simulink model "FieldControl_PID"  (R2021a)
settings: Solver=ode45  StartTime=0.0  StopTime=3  FixedStep=1e-5  MaxStep=1e-6  RelTol=1e-3
model workspace (MAT data in the model file):
  KI_s = 1
  KP_s = 1
undefined symbols (not defined in the file): DiscIntNeverNeededParam, Fsw, sigbuilder_block
libraries: simulink x2, spspowerguiLib x2
(part 2 of 2)

== system FieldControl_PID/Field_control_PID/Current_control/PMSM/Clark_Transformation ==
  Va : Inport
  Vb : Inport  Port=2
  Vc : Inport  Port=3
  Add : Sum  Inputs=+++
  Add1 : Sum
  Gain : Gain  Gain=-0.5
  Gain1 : Gain  Gain=-0.5
  Gain2 : Gain  Gain=2/3
  Gain3 : Gain  Gain=sqrt(3)/2
  Gain4 : Gain  Gain=-sqrt(3)/2
  Gain5 : Gain  Gain=2/3
  V_alpha : Outport
  V_beta : Outport  Port=2
  wires:
  Gain5/1 -> V_beta/1
  Add1/1 -> Gain5/1
  Gain3/1 -> Add1/1
  Gain4/1 -> Add1/2
  Gain2/1 -> V_alpha/1
  Add/1 -> Gain2/1
  Va/1 -> Add/1
  Gain1/1 -> Add/3
  Gain/1 -> Add/2
  Vc/1 -> Gain1/1, Gain4/1
  Vb/1 -> Gain/1, Gain3/1

== system FieldControl_PID/Field_control_PID/Current_control/PMSM/Electrical_system1 ==
  V_d : Inport
  V_q : Inport  Port=2
  W_e : Inport  Port=3
  Add : Sum  Inputs=-++
  Add1 : Sum  Inputs=+---
  Gain : Gain  Gain=1/Ld
  Gain1 : Gain  Gain=R/Ld
  Gain2 : Gain  Gain=Lq/Ld
  Gain3 : Gain  Gain=1/Lq
  Gain4 : Gain  Gain=R/Lq
  Gain5 : Gain  Gain=Ld/Lq
  Gain6 : Gain  Gain=lamda_pm/Lq
  Integrator : Integrator
  Integrator1 : Integrator
  Product : Product
  Product1 : Product
  I_d : Outport
  I_q : Outport  Port=2
  wires:
  Integrator/1 -> Gain5/1, Gain1/1, I_d/1
  Integrator1/1 -> Gain4/1, Gain2/1, I_q/1
  V_d/1 -> Gain/1
  Gain/1 -> Add/2
  Gain1/1 -> Add/1
  Add/1 -> Integrator/1
  Gain2/1 -> Product/2
  W_e/1 -> Product1/2, Gain6/1, Product/1
  Product/1 -> Add/3
  V_q/1 -> Gain3/1
  Gain3/1 -> Add1/1
  Gain4/1 -> Add1/4
  Gain5/1 -> Product1/1
  Product1/1 -> Add1/2
  Gain6/1 -> Add1/3
  Add1/1 -> Integrator1/1

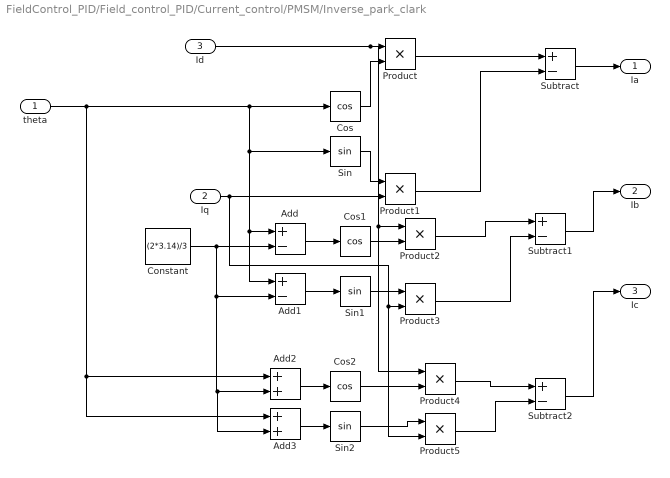
== system FieldControl_PID/Field_control_PID/Current_control/PMSM/Inverse_park_clark ==
  theta : Inport
  Iq : Inport  Port=2
  Id : Inport  Port=3
  Add : Sum  Inputs=+-
  Add1 : Sum  Inputs=+-
  Add2 : Sum
  Add3 : Sum
  Constant : Constant  Value=(2*3.14)/3
  Cos : Trigonometry  Operator=cos
  Cos1 : Trigonometry  Operator=cos
  Cos2 : Trigonometry  Operator=cos
  Product{,1..5} (6 alike) : Product
  Sin : Trigonometry
  Sin1 : Trigonometry
  Sin2 : Trigonometry
  Subtract : Sum  Inputs=+-
  Subtract1 : Sum  Inputs=+-
  Subtract2 : Sum  Inputs=+-
  Ia : Outport
  Ib : Outport  Port=2
  Ic : Outport  Port=3
  wires:
  Add3/1 -> Sin2/1
  Add2/1 -> Cos2/1
  Sin2/1 -> Product5/1
  Cos2/1 -> Product4/2
  Product5/1 -> Subtract2/2
  Product4/1 -> Subtract2/1
  Subtract2/1 -> Ic/1
  Constant/1 -> Add/2, Add1/2, Add2/2, Add3/2
  Subtract1/1 -> Ib/1
  Product3/1 -> Subtract1/2
  Product2/1 -> Subtract1/1
  Sin1/1 -> Product3/1
  Cos1/1 -> Product2/2
  Add1/1 -> Sin1/1
  Add/1 -> Cos1/1
  Product1/1 -> Subtract/2
  Sin/1 -> Product1/1
  Iq/1 -> Product1/2, Product3/2, Product5/2
  Product/1 -> Subtract/1
  Cos/1 -> Product/2
  Id/1 -> Product/1, Product2/1, Product4/1
  theta/1 -> Sin/1, Add/1, Add1/1, Cos/1, Add2/1, Add3/1
  Subtract/1 -> Ia/1

== system FieldControl_PID/Field_control_PID/Current_control/PMSM/Park_Transformation ==
  V_alpha : Inport
  V_beta : Inport  Port=2
  theta : Inport  Port=3
  Add : Sum
  Add1 : Sum
  Cos : Trigonometry  Operator=cos
  Cos1 : Trigonometry
  Gain : Gain  Gain=-1
  Product{,1..3} (4 alike) : Product
  V_d : Outport
  V_q : Outport  Port=2
  wires:
  Add1/1 -> V_q/1
  Product3/1 -> Add1/2
  Gain/1 -> Add1/1
  Product2/1 -> Gain/1
  Add/1 -> V_d/1
  Product1/1 -> Add/2
  Product/1 -> Add/1
  V_beta/1 -> Product1/2, Product3/1
  Cos1/1 -> Product1/1, Product2/2
  Cos/1 -> Product/2, Product3/2
  V_alpha/1 -> Product/1, Product2/1
  theta/1 -> Cos/1, Cos1/1

== system FieldControl_PID/Field_control_PID/Current_control/PMSM/Torque_system ==
  I_d : Inport
  I_q : Inport  Port=2
  Add : Sum  Inputs=+-
  Add1 : Sum
  Constant : Constant  Value=lamda_pm
  Gain : Gain  Gain=(3*P)/4
  Gain1 : Gain  Gain=Ld
  Gain2 : Gain  Gain=Lq
  Product : Product
  Product1 : Product
  Te : Outport
  wires:
  Product1/1 -> Add/2
  Gain2/1 -> Product1/2
  Product/1 -> Add/1
  I_q/1 -> Product/1, Gain2/1
  Add1/1 -> Product/2
  Gain1/1 -> Add1/1
  Constant/1 -> Add1/2
  I_d/1 -> Gain1/1, Product1/1
  Gain/1 -> Te/1
  Add/1 -> Gain/1

== system FieldControl_PID/Field_control_PID/Current_control/SVM-DPWM/Square_signal_generator ==
  Mode : Inport
  F : Inport  Port=2
  If : If  IfExpression=u1 == 1  ElseIfExpressions=u1==2  ShowElse=off
  If Action Subsystem : Subsystem  TreatAsAtomicUnit=on
  If Action Subsystem1 : Subsystem  TreatAsAtomicUnit=on
  Merge : Merge
  Output : Outport
  wires:
  Mode/1 -> If/1
  If/1 -> If Action Subsystem/Action
  F/1 -> If Action Subsystem1/1(F), If Action Subsystem/1(F)
  If/2 -> If Action Subsystem1/Action
  If Action Subsystem/1(out) -> Merge/1
  If Action Subsystem1/1(out) -> Merge/2
  Merge/1 -> Output/1

== system FieldControl_PID/Field_control_PID/Current_control/SVM-DPWM/Variant Subsystem ==
  note: 1) Add Subsystem or Model blocks as valid variant choices.
      | 2) You cannot connect blocks at this level. At simulation, connectivity is automatically
      | determined, based on the active variant and port name matching.
  Va : Inport
  Vb : Inport  Port=2
  Vc : Inport  Port=3
  Iabc : Inport  Port=4
  mag : Inport  Port=5
  Auto : Subsystem  VariantControl=PWM_Mode==3
  DPWM : Subsystem  VariantControl=PWM_Mode==2
  SVM : Subsystem  VariantControl=PWM_Mode==1
  V0 : Outport
  Va* : Outport  Port=2
  Vb* : Outport  Port=3
  Vc* : Outport  Port=4
  PWM_Gen_Mode : Outport  Port=5

== system FieldControl_PID/Field_control_PID/Current_control/Triggered Current Control/FFW ==
  Iq : Inport
  We : Inport  Port=2
  Id : Inport  Port=3
  Add : Sum
  Ld : Gain  Gain=0.0057
  Lq : Gain  Gain=0.0125
  Product : Product
  Product1 : Product
  "delta_pm " : Constant  Value=0.123
  Vq_FFW : Outport
  Vd_FFW : Outport  Port=2
  wires:
  "delta_pm "/1 -> Add/2
  Add/1 -> Product1/1
  Ld/1 -> Add/1
  Id/1 -> Ld/1
  Product1/1 -> Vq_FFW/1
  Product/1 -> Vd_FFW/1
  Lq/1 -> Product/2  "We*Lq"
  We/1 -> Lq/1, Product1/2
  Iq/1 -> Product/1  "Iq"

== system FieldControl_PID/Field_control_PID/Current_control/Triggered Current Control/PID_2 ==
  e : Inport
  Fsw_out : Inport  Port=2
  Discrete-Time Integrator : DiscreteIntegrator  SampleTime=-1  ICPrevOutput=DiscIntNeverNeededParam  ICPrevScaledInput=DiscIntNeverNeededParam
  Gain : Gain
  KI : Gain  Gain=1.2
  Kp : Gain  Gain=0.0125
  Product : Product
  Product1 : Product
  Scope : Scope
  Sum : Sum  Inputs=|++
  v : Outport
  wires:
  e/1 -> KI/1, Kp/1
  Discrete-Time Integrator/1 -> Scope/1, Sum/1
  Sum/1 -> v/1
  KI/1 -> Product/2
  Product/1 -> Discrete-Time Integrator/1
  Fsw_out/1 -> Gain/1
  Kp/1 -> Product1/2
  Product1/1 -> Sum/2
  Gain/1 -> Product1/1, Product/1

== system FieldControl_PID/Field_control_PID/Current_control/Triggered Current Control/PID_3 ==
  Fsw_out : Inport
  e : Inport  Port=2
  Discrete-Time Integrator : DiscreteIntegrator  SampleTime=-1  ICPrevOutput=DiscIntNeverNeededParam  ICPrevScaledInput=DiscIntNeverNeededParam
  Gain : Gain
  KI : Gain  Gain=1.2
  Kp : Gain  Gain=0.0057
  Product : Product
  Product1 : Product
  Sum : Sum  Inputs=|++
  v : Outport
  wires:
  Kp/1 -> Product1/2
  Product1/1 -> Sum/2
  KI/1 -> Product/2
  Product/1 -> Discrete-Time Integrator/1
  e/1 -> KI/1, Kp/1
  Sum/1 -> v/1
  Fsw_out/1 -> Gain/1
  Discrete-Time Integrator/1 -> Sum/1
  Gain/1 -> Product1/1, Product/1

== system FieldControl_PID/Field_control_PID/Current_control/Triggered Current Control/Signal Builder1 ==
  Demux : Demux  Tag=STV Demux  Outputs=1
      settings: DisplayOption=none
  FromWs : FromWorkspace  Tag=STV FromWs  VariableName=tuvar  SampleTime=-1
      SigBuilderData=|
      | common.afterFinalStr = 'Extrapolate'
      | common.sampleTime = '-1'
      | dataSet.timeRange = [0 3]
      | dataSet.name = 'Group 1'
      | sbobj.Groups.Name = 'Group 1'
      | sbobj.Groups.Signals.Name = 'Signal 1'
      | sbobj.Groups.Signals.XData = [0 1 1.5 2 2.5 3]
      | sbobj.Groups.Signals.YData = [2.5 2.5 3.5 3.5 5 5]
      | sbobj.Groups.TimeRange = [0 3]
  Signal 1 : Outport  Tag=STV Outport
  wires:
  Demux/1 -> Signal 1/1
  FromWs/1 -> Demux/1

== system FieldControl_PID/Field_control_PID/Speed_control/Inverse_park_clark/Subsystem ==
  Vd : Inport
  Vq : Inport  Port=2
  Add : Sum
  Square : Math  Operator=square  SaturateOnIntegerOverflow=on
  Square Root : Sqrt  SaturateOnIntegerOverflow=on
  Square1 : Math  Operator=square  SaturateOnIntegerOverflow=on
  Out1 : Outport
  wires:
  Square1/1 -> Add/1
  Add/1 -> Square Root/1
  Vd/1 -> Square1/1
  Square/1 -> Add/2
  Square Root/1 -> Out1/1
  Vq/1 -> Square/1

== system FieldControl_PID/Field_control_PID/Speed_control/PMSM/Clark_Transformation ==
  Va : Inport
  Vb : Inport  Port=2
  Vc : Inport  Port=3
  Add : Sum  Inputs=+++
  Add1 : Sum
  Gain : Gain  Gain=-0.5
  Gain1 : Gain  Gain=-0.5
  Gain2 : Gain  Gain=2/3
  Gain3 : Gain  Gain=sqrt(3)/2
  Gain4 : Gain  Gain=-sqrt(3)/2
  Gain5 : Gain  Gain=2/3
  V_alpha : Outport
  V_beta : Outport  Port=2
  wires:
  Gain5/1 -> V_beta/1
  Add1/1 -> Gain5/1
  Gain3/1 -> Add1/1
  Gain4/1 -> Add1/2
  Gain2/1 -> V_alpha/1
  Add/1 -> Gain2/1
  Va/1 -> Add/1
  Gain1/1 -> Add/3
  Gain/1 -> Add/2
  Vc/1 -> Gain1/1, Gain4/1
  Vb/1 -> Gain/1, Gain3/1

== system FieldControl_PID/Field_control_PID/Speed_control/PMSM/Electrical_system2 ==
  V_d : Inport
  V_q : Inport  Port=2
  W_e : Inport  Port=3
  Add : Sum  Inputs=-++
  Add1 : Sum  Inputs=+---
  Gain : Gain  Gain=1/Ld
  Gain1 : Gain  Gain=R/Ld
  Gain2 : Gain  Gain=Lq/Ld
  Gain3 : Gain  Gain=1/Lq
  Gain4 : Gain  Gain=R/Lq
  Gain5 : Gain  Gain=Ld/Lq
  Gain6 : Gain  Gain=lamda_pm/Lq
  Integrator : Integrator
  Integrator1 : Integrator
  Product : Product
  Product1 : Product
  I_d : Outport
  I_q : Outport  Port=2
  wires:
  Integrator/1 -> Gain5/1, Gain1/1, I_d/1
  Integrator1/1 -> Gain4/1, Gain2/1, I_q/1
  V_d/1 -> Gain/1
  Gain/1 -> Add/2
  Gain1/1 -> Add/1
  Add/1 -> Integrator/1
  Gain2/1 -> Product/2
  W_e/1 -> Gain6/1, Product1/2, Product/1
  Product/1 -> Add/3
  V_q/1 -> Gain3/1
  Gain3/1 -> Add1/1
  Gain4/1 -> Add1/4
  Gain5/1 -> Product1/1
  Product1/1 -> Add1/2
  Gain6/1 -> Add1/3
  Add1/1 -> Integrator1/1

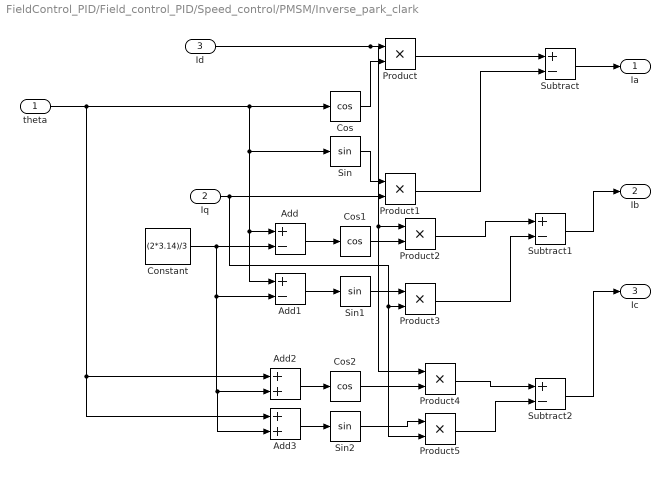
== system FieldControl_PID/Field_control_PID/Speed_control/PMSM/Inverse_park_clark ==
  theta : Inport
  Iq : Inport  Port=2
  Id : Inport  Port=3
  Add : Sum  Inputs=+-
  Add1 : Sum  Inputs=+-
  Add2 : Sum
  Add3 : Sum
  Constant : Constant  Value=(2*3.14)/3
  Cos : Trigonometry  Operator=cos
  Cos1 : Trigonometry  Operator=cos
  Cos2 : Trigonometry  Operator=cos
  Product{,1..5} (6 alike) : Product
  Sin : Trigonometry
  Sin1 : Trigonometry
  Sin2 : Trigonometry
  Subtract : Sum  Inputs=+-
  Subtract1 : Sum  Inputs=+-
  Subtract2 : Sum  Inputs=+-
  Ia : Outport
  Ib : Outport  Port=2
  Ic : Outport  Port=3
  wires:
  Add3/1 -> Sin2/1
  Add2/1 -> Cos2/1
  Sin2/1 -> Product5/1
  Cos2/1 -> Product4/2
  Product5/1 -> Subtract2/2
  Product4/1 -> Subtract2/1
  Subtract2/1 -> Ic/1
  Constant/1 -> Add/2, Add1/2, Add2/2, Add3/2
  Subtract1/1 -> Ib/1
  Product3/1 -> Subtract1/2
  Product2/1 -> Subtract1/1
  Sin1/1 -> Product3/1
  Cos1/1 -> Product2/2
  Add1/1 -> Sin1/1
  Add/1 -> Cos1/1
  Product1/1 -> Subtract/2
  Sin/1 -> Product1/1
  Iq/1 -> Product1/2, Product3/2, Product5/2
  Product/1 -> Subtract/1
  Cos/1 -> Product/2
  Id/1 -> Product/1, Product2/1, Product4/1
  theta/1 -> Sin/1, Add/1, Add1/1, Cos/1, Add2/1, Add3/1
  Subtract/1 -> Ia/1

== system FieldControl_PID/Field_control_PID/Speed_control/PMSM/Mechanical_system ==
  Te : Inport
  Add : Sum  Inputs=+--
  Add1 : Sum
  Gain : Gain  Gain=1/J
  Gain1 : Gain  Gain=1/J
  Gain2 : Gain  Gain=b/J
  Integrator : Integrator
  Step : Step  Time=1.2  Before=0.75  After=0.75  SampleTime=0
  Step1 : Step  Time=1.2  After=0.5  SampleTime=0
  TL : Constant  Value=TL
  Wm : Outport
  wires:
  Gain2/1 -> Add/3
  Gain/1 -> Add/1
  Add/1 -> Integrator/1
  Te/1 -> Gain/1
  Gain1/1 -> Add/2
  Integrator/1 -> Gain2/1, Wm/1
  Add1/1 -> Gain1/1
  Step/1 -> Add1/1
  Step1/1 -> Add1/2

== system FieldControl_PID/Field_control_PID/Speed_control/PMSM/Park_Transformation ==
  V_alpha : Inport
  V_beta : Inport  Port=2
  theta : Inport  Port=3
  Add : Sum
  Add1 : Sum
  Cos : Trigonometry  Operator=cos
  Cos1 : Trigonometry
  Gain : Gain  Gain=-1
  Product{,1..3} (4 alike) : Product
  V_d : Outport
  V_q : Outport  Port=2
  wires:
  Add1/1 -> V_q/1
  Product3/1 -> Add1/2
  Gain/1 -> Add1/1
  Product2/1 -> Gain/1
  Add/1 -> V_d/1
  Product1/1 -> Add/2
  Product/1 -> Add/1
  V_beta/1 -> Product1/2, Product3/1
  Cos1/1 -> Product1/1, Product2/2
  Cos/1 -> Product/2, Product3/2
  V_alpha/1 -> Product/1, Product2/1
  theta/1 -> Cos/1, Cos1/1

== system FieldControl_PID/Field_control_PID/Speed_control/PMSM/Torque_system ==
  I_d : Inport
  I_q : Inport  Port=2
  Add : Sum  Inputs=+-
  Add1 : Sum
  Constant : Constant  Value=lamda_pm
  Gain : Gain  Gain=(3*P)/4
  Gain1 : Gain  Gain=Ld
  Gain2 : Gain  Gain=Lq
  Product : Product
  Product1 : Product
  Te : Outport
  wires:
  Product1/1 -> Add/2
  Gain2/1 -> Product1/2
  Product/1 -> Add/1
  I_q/1 -> Product/1, Gain2/1
  Add1/1 -> Product/2
  Gain1/1 -> Add1/1
  Constant/1 -> Add1/2
  I_d/1 -> Gain1/1, Product1/1
  Gain/1 -> Te/1
  Add/1 -> Gain/1

== system FieldControl_PID/Field_control_PID/Speed_control/SVM-DPWM1/Square_signal_generator ==
  Mode : Inport
  F : Inport  Port=2
  If : If  IfExpression=u1 == 1  ElseIfExpressions=u1==2  ShowElse=off
  If Action Subsystem : Subsystem  TreatAsAtomicUnit=on
  If Action Subsystem1 : Subsystem  TreatAsAtomicUnit=on
  Merge : Merge
  Output : Outport
  wires:
  Mode/1 -> If/1
  If/1 -> If Action Subsystem/Action
  F/1 -> If Action Subsystem1/1(F), If Action Subsystem/1(F)
  If/2 -> If Action Subsystem1/Action
  If Action Subsystem/1(out) -> Merge/1
  If Action Subsystem1/1(out) -> Merge/2
  Merge/1 -> Output/1

== system FieldControl_PID/Field_control_PID/Speed_control/SVM-DPWM1/Variant Subsystem ==
  note: 1) Add Subsystem or Model blocks as valid variant choices.
      | 2) You cannot connect blocks at this level. At simulation, connectivity is automatically
      | determined, based on the active variant and port name matching.
  Va : Inport
  Vb : Inport  Port=2
  Vc : Inport  Port=3
  Iabc : Inport  Port=4
  mag : Inport  Port=5
  Auto : Subsystem  VariantControl=PWM_Mode==3
  DPWM : Subsystem  VariantControl=PWM_Mode==2
  SVM : Subsystem  VariantControl=PWM_Mode==1
  V0 : Outport
  Va* : Outport  Port=2
  Vb* : Outport  Port=3
  Vc* : Outport  Port=4
  PWM_Gen_Mode : Outport  Port=5

== system FieldControl_PID/Field_control_PID/Speed_control/Triggered Speed_Control/MTPA ==
  Tref : Inport
  MTPA_Eqns : Subsystem  VariantControl=Typee==1
  MTPA_Tables : Subsystem  VariantControl=Typee==2
  Id_ref : Outport
  Iq_ref : Outport  Port=2

== system FieldControl_PID/Field_control_PID/Speed_control/Triggered Speed_Control/PI_system3 ==
  Error : Inport
  AND : Logic  Operator=NAND  AllPortsSameDT=off  OutDataTypeStr=boolean
  Discrete-Time Integrator : DiscreteIntegrator  SampleTime=-1  ICPrevOutput=DiscIntNeverNeededParam  ICPrevScaledInput=DiscIntNeverNeededParam
  Equal : RelationalOperator  Operator=~=  OutDataTypeStr=boolean  RndMeth=Simplest
  Equal1 : RelationalOperator  Operator===  OutDataTypeStr=boolean  RndMeth=Simplest
  KI : Gain  Gain=5
  Kp : Gain  Gain=0.05
  Product : Product
  Saturation1 : Saturate  UpperLimit=1.59  LowerLimit=0
  Sign : Signum
  Sign1 : Signum
  Sum : Sum  Inputs=|++
  Unit Delay : UnitDelay  SampleTime=-1  HasFrameUpgradeWarning=on
  Unit Delay1 : UnitDelay  SampleTime=-1  HasFrameUpgradeWarning=on
  T_ref : Outport
  wires:
  Error/1 -> Kp/1, Sign1/1, Product/2
  AND/1 -> Product/1
  Unit Delay1/1 -> Equal/2
  Product/1 -> KI/1
  Unit Delay/1 -> Equal/1, Sign/1
  Equal/1 -> AND/2
  Equal1/1 -> AND/1
  Sign1/1 -> Equal1/1
  Sign/1 -> Equal1/2
  Saturation1/1 -> Unit Delay1/1, T_ref/1
  Sum/1 -> Saturation1/1, Unit Delay/1
  KI/1 -> Discrete-Time Integrator/1
  Kp/1 -> Sum/2
  Discrete-Time Integrator/1 -> Sum/1

== system FieldControl_PID/Field_control_PID/Speed_control/Triggered Speed_Control/Signal Builder2 ==
  Demux : Demux  Tag=STV Demux  Outputs=1
      settings: DisplayOption=none
  FromWs : FromWorkspace  Tag=STV FromWs  VariableName=tuvar  SampleTime=-1
      SigBuilderData=|
      | common.afterFinalStr = 'Extrapolate'
      | common.sampleTime = '-1'
      | dataSet.timeRange = [0 3]
      | dataSet.name = 'Group 1'
      | sbobj.Groups.Name = 'Group 1'
      | sbobj.Groups.Signals.Name = 'Signal 1'
      | sbobj.Groups.Signals.XData = [0 0.25 0.5 1 1.5 1.75 2 2.5 2.75 3]
      | sbobj.Groups.Signals.YData = [0 0.5 0.5 1.5 1.5 2 1.5 1.5 0.5 0.5]
      | sbobj.Groups.TimeRange = [0 3]
  Signal 1 : Outport  Tag=STV Outport
  wires:
  FromWs/1 -> Demux/1
  Demux/1 -> Signal 1/1

== system FieldControl_PID/Field_control_PID/Speed_control/Triggered Speed_Control/Some_Edits ==
  1-D Lookup Id : Lookup_n-D  Commented=on  NumberOfTableDimensions=1  BreakpointsForDimension1=[0.1,0.15,0.2,0.25,0.3,0.35,0.4,0.45,0.5,0.55,0.6,0.65,0.7,0.75,0.8,0.85,0.9,0.95,1,1.05,1.1,1.15,1.2,1.25,1.3,1.35,1.4,1.45,1.5,1.55]  Table=[-0.0672,-0.2941,-0.0672,-0.2027,-0.0672,-0.1637,-0.0672,-0.1422,-0.0672,-0.1285,-0.1799,-0.119,-0.1637,-0.2027,-0.2369,-0.2671,-0.2941,-0.3183,-0.4097,-0.4264,-0.4415,-0.5166,-0.5268,-0.593,-0.5996,-0.6586,-1.2981,-1.9904,-2.6828,-3.3752]  InternalRulePriority=Speed  RndMeth=Simplest  InputSameDT=on
  1-D Lookup Iq : Lookup_n-D  Commented=on  NumberOfTableDimensions=1  BreakpointsForDimension1=[0.1,0.15,0.2,0.25,0.3,0.35,0.4,0.45,0.5,0.55,0.6,0.65,0.7,0.75,0.8,0.85,0.9,0.95,1,1.05,1.1,1.15,1.2,1.25,1.3,1.35,1.4,1.45,1.5,1.55]  Table=[0.27,0.4,0.54,0.67,0.81,0.94,1.08,1.21,1.35,1.48,1.61,1.75,1.88,2.01,2.14,2.27,2.4,2.53,2.65,2.78,2.91,3.03,3.16,3.28,3.41,3.53,3.54,3.54,3.54,3.54]  InternalRulePriority=Speed  RndMeth=Simplest  InputSameDT=on
  1-D Lookup Table2 : Lookup_n-D  Commented=on  NumberOfTableDimensions=1  BreakpointsForDimension1=|  Table=|  InternalRulePriority=Speed  RndMeth=Simplest  InputSameDT=on
      BreakpointsForDimension1=|
      | [ 0.16
      | 0.26
      | 0.36
      | 0.46
      | 0.56
      | 0.66
      | 0.76
      | 0.86
      | 0.96
      | 1.06
      | 1.16
      | 1.26
      | 1.36
      | 1.46
      | 1.56
      | ]
      Table=|
      | [
      |  2.401960784
      | 1.094771242
      | 0.441176471
      | 0.049019608
      | -0.212418301
      | -0.399159664
      | -0.539215686
      | -0.648148148
      | -0.735294118
      | -0.806595365
      | -0.866013072
      | -0.916289593
      | -0.959383754
      | -1.654834348
      | -3.007099391
      | ]
  1-D Lookup Table3 : Lookup_n-D  Commented=on  NumberOfTableDimensions=1  BreakpointsForDimension1=[0.16 0.26 0.36 0.46 0.56 0.66 0.76 0.86 0.96 1.06 1.16 1.26 1.36 1.46 1.56]  Table=|  InternalRulePriority=Speed  RndMeth=Simplest  InputSameDT=on
      | [
      | 0.5
      | 
      | 0.75
      | 
      | 1
      | 
      | 1.25
      | 
      | 1.5
      | 
      | 1.75
      | 
      | 2
      | 
      | 2.25
      | 
      | 2.5
      | 
      | 2.75
      | 
      | 3
      | 
      | 3.25
      | 3.5
      | 3.625 
      | 3.625]
  Add1 : Sum  Commented=on
  PI_system2 : Subsystem  Commented=on
  Step3 : Step  Commented=on  Time=2  After=100  SampleTime=0
  Step4 : Step  Commented=on  Before=200  After=250  SampleTime=0
  Subsystem : Subsystem  Commented=on
  wires:
  Step4/1 -> Add1/1
  Step3/1 -> Add1/2

== system FieldControl_PID/Field_control_PID/Speed_control/Triggered Speed_Control/Switching_Frequency ==
  Wm : Inport
  Chart : Stateflow chart  TreatAsAtomicUnit=on
  Constant1 : Constant  Value=Lower_Limit
  Constant3 : Constant  Value=Higher_Limit
  Gain : Gain  Gain=1/500
  Gain1 : Gain  Gain=500
  Gain2 : Gain  Gain=Sw2fund_Ration
  N2F : Gain  Gain=4/120
  Round : Rounding  Operator=round
  Wm2N : Gain  Gain=60/(2*pi)
  Fsw_out : Outport
  Sampling_Mode : Outport  Port=2
  wires:
  Wm/1 -> Wm2N/1
  N2F/1 -> Gain2/1
  Gain2/1 -> Chart/3(Fsw_input)
  Chart/2(Sampling_Mode) -> Sampling_Mode/1
  Constant3/1 -> Chart/2(High_Limit)
  Constant1/1 -> Chart/1(Low_limit)
  Wm2N/1 -> N2F/1
  Chart/1(Fsw_out) -> Gain/1
  Gain/1 -> Round/1
  Round/1 -> Gain1/1
  Gain1/1 -> Fsw_out/1

== system FieldControl_PID/Field_control_PID/Speed_control/Triggered Subsystem/FFW ==
  Iq : Inport
  We : Inport  Port=2
  Id : Inport  Port=3
  Add : Sum
  Ld : Gain  Gain=0.0057
  Lq : Gain  Gain=0.0125
  Product : Product
  Product1 : Product
  "delta_pm " : Constant  Value=0.123
  Vq_FFW : Outport
  Vd_FFW : Outport  Port=2
  wires:
  "delta_pm "/1 -> Add/2
  Add/1 -> Product1/1
  Ld/1 -> Add/1
  Id/1 -> Ld/1
  Product1/1 -> Vq_FFW/1
  Product/1 -> Vd_FFW/1
  Lq/1 -> Product/2  "We*Lq"
  We/1 -> Lq/1, Product1/2
  Iq/1 -> Product/1  "Iq"

== system FieldControl_PID/Field_control_PID/Speed_control/Triggered Subsystem/PID_2 ==
  e : Inport
  Fsw_out : Inport  Port=2
  Discrete-Time Integrator : DiscreteIntegrator  SampleTime=-1  ICPrevOutput=DiscIntNeverNeededParam  ICPrevScaledInput=DiscIntNeverNeededParam
  Gain : Gain
  KI : Gain  Gain=1.2
  Kp : Gain  Gain=0.0125
  Product : Product
  Product1 : Product
  Scope : Scope
  Sum : Sum  Inputs=|++
  v : Outport
  wires:
  e/1 -> KI/1, Kp/1
  Discrete-Time Integrator/1 -> Scope/1, Sum/1
  Sum/1 -> v/1
  KI/1 -> Product/2
  Product/1 -> Discrete-Time Integrator/1
  Fsw_out/1 -> Gain/1
  Kp/1 -> Product1/2
  Product1/1 -> Sum/2
  Gain/1 -> Product1/1, Product/1

== system FieldControl_PID/Field_control_PID/Speed_control/Triggered Subsystem/PID_3 ==
  Fsw_out : Inport
  e : Inport  Port=2
  Discrete-Time Integrator : DiscreteIntegrator  SampleTime=-1  ICPrevOutput=DiscIntNeverNeededParam  ICPrevScaledInput=DiscIntNeverNeededParam
  Gain : Gain
  KI : Gain  Gain=1.2
  Kp : Gain  Gain=0.0057
  Product : Product
  Product1 : Product
  Sum : Sum  Inputs=|++
  v : Outport
  wires:
  Kp/1 -> Product1/2
  Product1/1 -> Sum/2
  KI/1 -> Product/2
  Product/1 -> Discrete-Time Integrator/1
  e/1 -> KI/1, Kp/1
  Sum/1 -> v/1
  Fsw_out/1 -> Gain/1
  Discrete-Time Integrator/1 -> Sum/1
  Gain/1 -> Product1/1, Product/1

== system FieldControl_PID/Field_control_PID/Current_control/SVM-DPWM/Square_signal_generator/If Action Subsystem ==
  F : Inport
  Action Port : ActionPort  ActionPortLabel=if(u1 == 1 )
  Abs : Abs
  Clock1 : Clock
  Constant2 : Constant
  Constant3 : Constant  Value=0.5
  Constant4 : Constant
  Divide : Product  Inputs=**
  Gain : Gain  Gain=0.5
  Gain1 : Gain  Gain=4
  Mod1 : Math  Operator=mod  SaturateOnIntegerOverflow=on
  Subtract : Sum  Inputs=+-
  Subtract1 : Sum  Inputs=+-
  out : Outport
  wires:
  Constant4/1 -> Subtract1/2
  Mod1/1 -> Subtract/1
  Divide/1 -> Mod1/1
  Constant2/1 -> Mod1/2
  Subtract1/1 -> out/1
  Subtract/1 -> Abs/1
  Abs/1 -> Gain1/1
  Clock1/1 -> Divide/1
  Gain1/1 -> Subtract1/1
  Constant3/1 -> Subtract/2
  F/1 -> Gain/1
  Gain/1 -> Divide/2

== system FieldControl_PID/Field_control_PID/Current_control/SVM-DPWM/Square_signal_generator/If Action Subsystem1 ==
  F : Inport
  Action Port : ActionPort  ActionPortLabel=elseif( u1==2)
  Abs : Abs
  Clock1 : Clock
  Constant2 : Constant
  Constant3 : Constant  Value=0.5
  Constant4 : Constant
  Divide : Product  Inputs=**
  Gain1 : Gain  Gain=4
  Mod1 : Math  Operator=mod  SaturateOnIntegerOverflow=on
  Subtract : Sum  Inputs=+-
  Subtract1 : Sum  Inputs=+-
  out : Outport
  wires:
  F/1 -> Divide/2
  Gain1/1 -> Subtract1/1
  Clock1/1 -> Divide/1
  Constant3/1 -> Subtract/2
  Subtract/1 -> Abs/1
  Subtract1/1 -> out/1
  Constant4/1 -> Subtract1/2
  Mod1/1 -> Subtract/1
  Abs/1 -> Gain1/1
  Divide/1 -> Mod1/1
  Constant2/1 -> Mod1/2

== system FieldControl_PID/Field_control_PID/Current_control/SVM-DPWM/Variant Subsystem/Auto ==
  Iabc : Inport
  Va : Inport  Port=2
  Vb : Inport  Port=3
  Vc : Inport  Port=4
  mag : Inport  Port=5
  Compare To Constant : simulink/Logic and Bit Operations/Compare To Constant  relop=>  const=0.5  OutDataTypeStr=boolean
  Gain : Gain  Gain=sqrt(3)/Vdc
  If : If  IfExpression=u1 > 0.5
  If Action Subsystem : Subsystem  TreatAsAtomicUnit=on
  If Action Subsystem1 : Subsystem  TreatAsAtomicUnit=on
  Merge : Merge
  Scope : Scope
  Va* : Outport
  Vb* : Outport  Port=2
  Vc* : Outport  Port=3
  V0 : Outport  Port=4
  PWM_Gen_Mode : Outport  Port=5
  wires:
  Va/1 -> Va*/1, If Action Subsystem1/1(Va1), If Action Subsystem/1(Va1)
  Vb/1 -> Vb*/1, If Action Subsystem1/2(Vb1), If Action Subsystem/2(Vb1)
  Vc/1 -> Vc*/1, If Action Subsystem1/3(Vc1), If Action Subsystem/3(Vc1)
  Iabc/1 -> If Action Subsystem1/4(Iabc)
  If Action Subsystem/1(V1) -> Merge/1
  If Action Subsystem1/1(V1) -> Merge/2
  Merge/1 -> V0/1
  If/1 -> If Action Subsystem1/Action
  If/2 -> If Action Subsystem/Action
  Gain/1 -> Compare To Constant/1, Scope/1, If/1
  mag/1 -> Gain/1
  Compare To Constant/1 -> PWM_Gen_Mode/1

== system FieldControl_PID/Field_control_PID/Current_control/SVM-DPWM/Variant Subsystem/DPWM ==
  Va : Inport
  Vb : Inport  Port=2
  Vc : Inport  Port=3
  Iabc : Inport  Port=4
  Abs3 : Abs
  Abs4 : Abs
  Abs5 : Abs
  Constant : Constant
  Demux : Demux  Outputs=3
  Gain : Gain  Gain=1/5
  MATLAB Function1 : MATLAB Function  TreatAsAtomicUnit=on
  Max1 : MinMax  Function=max  Inputs=3
  Scope : Scope
  Sum1 : Sum  Inputs=|-+
  Va* : Outport
  Vb* : Outport  Port=2
  Vc* : Outport  Port=3
  V0 : Outport  Port=4
  PWM_Gen_Mode : Outport  Port=5
  wires:
  Gain/1 -> Demux/1
  Abs5/1 -> Max1/3
  MATLAB Function1/2(y) -> Sum1/2
  Abs3/1 -> Max1/1
  Abs4/1 -> Max1/2
  Max1/1 -> MATLAB Function1/7(max_i)  "max_i"
  MATLAB Function1/1(x) -> Sum1/1
  Va/1 -> Va*/1, MATLAB Function1/1(va)  "va"
  Vb/1 -> Vb*/1, MATLAB Function1/2(vb)  "vb"
  Vc/1 -> Vc*/1, MATLAB Function1/3(vc)  "vc"
  Iabc/1 -> Gain/1
  Demux/1 -> Abs3/1, MATLAB Function1/4(ia)
  Demux/2 -> Abs4/1, MATLAB Function1/5(ib)
  Demux/3 -> Abs5/1, MATLAB Function1/6(ic)
  Sum1/1 -> Scope/1, V0/1  "zero_seq"
  Constant/1 -> PWM_Gen_Mode/1

== system FieldControl_PID/Field_control_PID/Current_control/SVM-DPWM/Variant Subsystem/SVM ==
  Va : Inport
  Vb : Inport  Port=2
  Vc : Inport  Port=3
  Iabc : Inport  Port=4
  Add : Sum
  Constant : Constant  Value=0
  Gain : Gain  Gain=-1/2
  Max : MinMax  Function=max  Inputs=3
  Max1 : MinMax  Inputs=3
  Terminator : Terminator
  V0 : Outport
  Va* : Outport  Port=2
  Vb* : Outport  Port=3
  Vc* : Outport  Port=4
  PWM_Gen_Mode : Outport  Port=5
  wires:
  Gain/1 -> V0/1
  Vc/1 -> Vc*/1, Max1/3, Max/3
  Vb/1 -> Vb*/1, Max1/2, Max/2
  Max/1 -> Add/1
  Max1/1 -> Add/2
  Add/1 -> Gain/1
  Va/1 -> Va*/1, Max1/1, Max/1
  Iabc/1 -> Terminator/1
  Constant/1 -> PWM_Gen_Mode/1

== system FieldControl_PID/Field_control_PID/Speed_control/SVM-DPWM1/Square_signal_generator/If Action Subsystem ==
  F : Inport
  Action Port : ActionPort  ActionPortLabel=if(u1 == 1 )
  Abs : Abs
  Clock1 : Clock
  Constant2 : Constant
  Constant3 : Constant  Value=0.5
  Constant4 : Constant
  Divide : Product  Inputs=**
  Gain : Gain  Gain=0.5
  Gain1 : Gain  Gain=4
  Mod1 : Math  Operator=mod  SaturateOnIntegerOverflow=on
  Subtract : Sum  Inputs=+-
  Subtract1 : Sum  Inputs=+-
  out : Outport
  wires:
  Constant4/1 -> Subtract1/2
  Mod1/1 -> Subtract/1
  Divide/1 -> Mod1/1
  Constant2/1 -> Mod1/2
  Subtract1/1 -> out/1
  Subtract/1 -> Abs/1
  Abs/1 -> Gain1/1
  Clock1/1 -> Divide/1
  Gain1/1 -> Subtract1/1
  Constant3/1 -> Subtract/2
  F/1 -> Gain/1
  Gain/1 -> Divide/2

== system FieldControl_PID/Field_control_PID/Speed_control/SVM-DPWM1/Square_signal_generator/If Action Subsystem1 ==
  F : Inport
  Action Port : ActionPort  ActionPortLabel=elseif( u1==2)
  Abs : Abs
  Clock1 : Clock
  Constant2 : Constant
  Constant3 : Constant  Value=0.5
  Constant4 : Constant
  Divide : Product  Inputs=**
  Gain1 : Gain  Gain=4
  Mod1 : Math  Operator=mod  SaturateOnIntegerOverflow=on
  Subtract : Sum  Inputs=+-
  Subtract1 : Sum  Inputs=+-
  out : Outport
  wires:
  F/1 -> Divide/2
  Gain1/1 -> Subtract1/1
  Clock1/1 -> Divide/1
  Constant3/1 -> Subtract/2
  Subtract/1 -> Abs/1
  Subtract1/1 -> out/1
  Constant4/1 -> Subtract1/2
  Mod1/1 -> Subtract/1
  Abs/1 -> Gain1/1
  Divide/1 -> Mod1/1
  Constant2/1 -> Mod1/2

== system FieldControl_PID/Field_control_PID/Speed_control/SVM-DPWM1/Variant Subsystem/Auto ==
  Iabc : Inport
  Va : Inport  Port=2
  Vb : Inport  Port=3
  Vc : Inport  Port=4
  mag : Inport  Port=5
  Compare To Constant : simulink/Logic and Bit Operations/Compare To Constant  relop=>  const=0.5  OutDataTypeStr=boolean
  Gain : Gain  Gain=sqrt(3)/Vdc
  If : If  IfExpression=u1 > 0.5
  If Action Subsystem : Subsystem  TreatAsAtomicUnit=on
  If Action Subsystem1 : Subsystem  TreatAsAtomicUnit=on
  Merge : Merge
  Scope : Scope
  Va* : Outport
  Vb* : Outport  Port=2
  Vc* : Outport  Port=3
  V0 : Outport  Port=4
  PWM_Gen_Mode : Outport  Port=5
  wires:
  Va/1 -> Va*/1, If Action Subsystem1/1(Va1), If Action Subsystem/1(Va1)
  Vb/1 -> Vb*/1, If Action Subsystem1/2(Vb1), If Action Subsystem/2(Vb1)
  Vc/1 -> Vc*/1, If Action Subsystem1/3(Vc1), If Action Subsystem/3(Vc1)
  Iabc/1 -> If Action Subsystem1/4(Iabc)
  If Action Subsystem/1(V1) -> Merge/1
  If Action Subsystem1/1(V1) -> Merge/2
  Merge/1 -> V0/1
  If/1 -> If Action Subsystem1/Action
  If/2 -> If Action Subsystem/Action
  Gain/1 -> Compare To Constant/1, Scope/1, If/1
  mag/1 -> Gain/1
  Compare To Constant/1 -> PWM_Gen_Mode/1

== system FieldControl_PID/Field_control_PID/Speed_control/SVM-DPWM1/Variant Subsystem/DPWM ==
  Va : Inport
  Vb : Inport  Port=2
  Vc : Inport  Port=3
  Iabc : Inport  Port=4
  Abs3 : Abs
  Abs4 : Abs
  Abs5 : Abs
  Constant : Constant
  Demux : Demux  Outputs=3
  Gain : Gain  Gain=1/5
  MATLAB Function1 : MATLAB Function  TreatAsAtomicUnit=on
  Max1 : MinMax  Function=max  Inputs=3
  Scope : Scope
  Sum1 : Sum  Inputs=|-+
  Va* : Outport
  Vb* : Outport  Port=2
  Vc* : Outport  Port=3
  V0 : Outport  Port=4
  PWM_Gen_Mode : Outport  Port=5
  wires:
  Gain/1 -> Demux/1
  Abs5/1 -> Max1/3
  MATLAB Function1/2(y) -> Sum1/2
  Abs3/1 -> Max1/1
  Abs4/1 -> Max1/2
  Max1/1 -> MATLAB Function1/7(max_i)  "max_i"
  MATLAB Function1/1(x) -> Sum1/1
  Va/1 -> Va*/1, MATLAB Function1/1(va)  "va"
  Vb/1 -> Vb*/1, MATLAB Function1/2(vb)  "vb"
  Vc/1 -> Vc*/1, MATLAB Function1/3(vc)  "vc"
  Iabc/1 -> Gain/1
  Demux/1 -> Abs3/1, MATLAB Function1/4(ia)
  Demux/2 -> Abs4/1, MATLAB Function1/5(ib)
  Demux/3 -> Abs5/1, MATLAB Function1/6(ic)
  Sum1/1 -> Scope/1, V0/1  "zero_seq"
  Constant/1 -> PWM_Gen_Mode/1

== system FieldControl_PID/Field_control_PID/Speed_control/SVM-DPWM1/Variant Subsystem/SVM ==
  Va : Inport
  Vb : Inport  Port=2
  Vc : Inport  Port=3
  Iabc : Inport  Port=4
  Add : Sum
  Constant : Constant  Value=0
  Gain : Gain  Gain=-1/2
  Max : MinMax  Function=max  Inputs=3
  Max1 : MinMax  Inputs=3
  Terminator : Terminator
  V0 : Outport
  Va* : Outport  Port=2
  Vb* : Outport  Port=3
  Vc* : Outport  Port=4
  PWM_Gen_Mode : Outport  Port=5
  wires:
  Gain/1 -> V0/1
  Vc/1 -> Vc*/1, Max1/3, Max/3
  Vb/1 -> Vb*/1, Max1/2, Max/2
  Max/1 -> Add/1
  Max1/1 -> Add/2
  Add/1 -> Gain/1
  Va/1 -> Va*/1, Max1/1, Max/1
  Iabc/1 -> Terminator/1
  Constant/1 -> PWM_Gen_Mode/1

== system FieldControl_PID/Field_control_PID/Speed_control/Triggered Speed_Control/MTPA/MTPA_Eqns ==
  Tref : Inport
  Add : Sum
  Constant : Constant  Value=0.123/(4*(0.0125-0.0057))
  Constant1 : Constant  Value=((0.123)^2)/(16*((0.0125-0.0057)^2))
  Gain : Gain  Gain=2/(3*2*0.123)
  Gain1 : Gain  Gain=0.5
  IMAX : Constant  Value=5
  Min : MinMax  Inputs=2
  Sqrt : Sqrt  SaturateOnIntegerOverflow=on
  Sqrt1 : Sqrt  SaturateOnIntegerOverflow=on
  Square : Math  Operator=square  SaturateOnIntegerOverflow=on
  Square1 : Math  Operator=square  SaturateOnIntegerOverflow=on
  Subtract : Sum  Inputs=+-
  Subtract1 : Sum  Inputs=+-
  Id_ref : Outport
  Iq_ref : Outport  Port=2
  wires:
  Min/1 -> Square/1  "Im"
  IMAX/1 -> Min/1
  Gain/1 -> Min/2  "Im"
  Square1/1 -> Subtract1/2
  Add/1 -> Sqrt/1
  Subtract1/1 -> Sqrt1/1
  Subtract/1 -> Id_ref/1, Square1/1
  Sqrt/1 -> Subtract/2
  Tref/1 -> Gain/1
  Gain1/1 -> Add/2
  Constant1/1 -> Add/1
  Square/1 -> Gain1/1, Subtract1/1
  Sqrt1/1 -> Iq_ref/1
  Constant/1 -> Subtract/1

== system FieldControl_PID/Field_control_PID/Speed_control/Triggered Speed_Control/MTPA/MTPA_Tables ==
  Tref : Inport
  1-D Lookup Id : Lookup_n-D  NumberOfTableDimensions=1  BreakpointsForDimension1=[0.1,0.15,0.2,0.25,0.3,0.35,0.4,0.45,0.5,0.55,0.6,0.65,0.7,0.75,0.8,0.85,0.9,0.95,1,1.05,1.1,1.15,1.2,1.25,1.3,1.35,1.4,1.45,1.5,1.55]  Table=[-0.0672,-0.2941,-0.0672,-0.2027,-0.0672,-0.1637,-0.0672,-0.1422,-0.0672,-0.1285,-0.1799,-0.119,-0.1637,-0.2027,-0.2369,-0.2671,-0.2941,-0.3183,-0.4097,-0.4264,-0.4415,-0.5166,-0.5268,-0.593,-0.5996,-0.6586,-1.2981,-1.9904,-2.6828,-3.3752]  InternalRulePriority=Speed  RndMeth=Simplest  InputSameDT=on
  1-D Lookup Iq : Lookup_n-D  NumberOfTableDimensions=1  BreakpointsForDimension1=[0.1,0.15,0.2,0.25,0.3,0.35,0.4,0.45,0.5,0.55,0.6,0.65,0.7,0.75,0.8,0.85,0.9,0.95,1,1.05,1.1,1.15,1.2,1.25,1.3,1.35,1.4,1.45,1.5,1.55]  Table=[0.27,0.4,0.54,0.67,0.81,0.94,1.08,1.21,1.35,1.48,1.61,1.75,1.88,2.01,2.14,2.27,2.4,2.53,2.65,2.78,2.91,3.03,3.16,3.28,3.41,3.53,3.54,3.54,3.54,3.54]  InternalRulePriority=Speed  RndMeth=Simplest  InputSameDT=on
  Id_ref : Outport
  Iq_ref : Outport  Port=2
  wires:
  1-D Lookup Iq/1 -> Iq_ref/1  "Iq"
  1-D Lookup Id/1 -> Id_ref/1  "Id"
  Tref/1 -> 1-D Lookup Id/1, 1-D Lookup Iq/1

== system FieldControl_PID/Field_control_PID/Speed_control/Triggered Speed_Control/Some_Edits/PI_system2 ==
  In1 : Inport
  Discrete-Time Integrator : DiscreteIntegrator  SampleTime=10/Fsw  ICPrevOutput=DiscIntNeverNeededParam  ICPrevScaledInput=DiscIntNeverNeededParam
  KI : Gain  Gain=3.12
  Kp : Gain  Gain=19.5
  Saturation1 : Saturate  UpperLimit=1.6  LowerLimit=0
  Sum : Sum  Inputs=|++
  T_ref : Outport
  wires:
  Saturation1/1 -> T_ref/1
  Sum/1 -> Saturation1/1
  In1/1 -> KI/1, Kp/1
  KI/1 -> Discrete-Time Integrator/1
  Kp/1 -> Sum/2
  Discrete-Time Integrator/1 -> Sum/1

== system FieldControl_PID/Field_control_PID/Speed_control/Triggered Speed_Control/Some_Edits/Subsystem ==
  Tref : Inport
  Add : Sum
  Constant : Constant  Value=0.123/(4*(0.0125-0.0057))
  Constant1 : Constant  Value=((0.123)^2)/(16*((0.0125-0.0057)^2))
  Gain : Gain  Gain=2/(3*2*0.123)
  Gain1 : Gain  Gain=0.5
  Scope : Scope
  Sqrt : Sqrt  SaturateOnIntegerOverflow=on
  Sqrt1 : Sqrt  SaturateOnIntegerOverflow=on
  Square : Math  Operator=square  SaturateOnIntegerOverflow=on
  Square1 : Math  Operator=square  SaturateOnIntegerOverflow=on
  Subtract : Sum  Inputs=+-
  Subtract1 : Sum  Inputs=+-
  Id_ref : Outport
  Iq_ref : Outport  Port=2
  wires:
  Sqrt1/1 -> Iq_ref/1
  Subtract1/1 -> Sqrt1/1
  Square1/1 -> Subtract1/2
  Gain1/1 -> Add/2
  Square/1 -> Gain1/1, Subtract1/1
  Constant1/1 -> Add/1
  Subtract/1 -> Id_ref/1, Square1/1
  Sqrt/1 -> Subtract/2
  Add/1 -> Sqrt/1
  Constant/1 -> Subtract/1
  Gain/1 -> Square/1, Scope/1  "Im"
  Tref/1 -> Gain/1

== system FieldControl_PID/Field_control_PID/Current_control/SVM-DPWM/Variant Subsystem/Auto/If Action Subsystem ==
  Va1 : Inport
  Vb1 : Inport  Port=2
  Vc1 : Inport  Port=3
  Action Port : ActionPort  ActionPortLabel=else
  Add : Sum
  Gain1 : Gain  Gain=-1/2
  Max : MinMax  Function=max  Inputs=3
  Max2 : MinMax  Inputs=3
  V1 : Outport
  wires:
  Add/1 -> Gain1/1
  Max2/1 -> Add/2
  Max/1 -> Add/1
  Va1/1 -> Max2/1, Max/1
  Vb1/1 -> Max2/2, Max/2
  Vc1/1 -> Max2/3, Max/3
  Gain1/1 -> V1/1

== system FieldControl_PID/Field_control_PID/Current_control/SVM-DPWM/Variant Subsystem/Auto/If Action Subsystem1 ==
  Va1 : Inport
  Vb1 : Inport  Port=2
  Vc1 : Inport  Port=3
  Iabc : Inport  Port=4
  Action Port : ActionPort  ActionPortLabel=if(u1 > 0.5)
  Abs3 : Abs
  Abs4 : Abs
  Abs5 : Abs
  Demux : Demux  Outputs=3
  Gain : Gain  Gain=1/5
  MATLAB Function1 : MATLAB Function  TreatAsAtomicUnit=on
  Max1 : MinMax  Function=max  Inputs=3
  Sum1 : Sum  Inputs=|-+
  V1 : Outport
  wires:
  Abs3/1 -> Max1/1
  MATLAB Function1/2(y) -> Sum1/2
  Gain/1 -> Demux/1
  MATLAB Function1/1(x) -> Sum1/1
  Abs4/1 -> Max1/2
  Abs5/1 -> Max1/3
  Max1/1 -> MATLAB Function1/7(max_i)  "max_i"
  Demux/3 -> MATLAB Function1/6(ic), Abs5/1
  Demux/2 -> MATLAB Function1/5(ib), Abs4/1
  Demux/1 -> MATLAB Function1/4(ia), Abs3/1
  Sum1/1 -> V1/1  "zero_seq"
  Va1/1 -> MATLAB Function1/1(va)
  Vb1/1 -> MATLAB Function1/2(vb)
  Vc1/1 -> MATLAB Function1/3(vc)
  Iabc/1 -> Gain/1

== system FieldControl_PID/Field_control_PID/Speed_control/SVM-DPWM1/Variant Subsystem/Auto/If Action Subsystem ==
  Va1 : Inport
  Vb1 : Inport  Port=2
  Vc1 : Inport  Port=3
  Action Port : ActionPort  ActionPortLabel=else
  Add : Sum
  Gain1 : Gain  Gain=-1/2
  Max : MinMax  Function=max  Inputs=3
  Max2 : MinMax  Inputs=3
  V1 : Outport
  wires:
  Add/1 -> Gain1/1
  Max2/1 -> Add/2
  Max/1 -> Add/1
  Va1/1 -> Max2/1, Max/1
  Vb1/1 -> Max2/2, Max/2
  Vc1/1 -> Max2/3, Max/3
  Gain1/1 -> V1/1

== system FieldControl_PID/Field_control_PID/Speed_control/SVM-DPWM1/Variant Subsystem/Auto/If Action Subsystem1 ==
  Va1 : Inport
  Vb1 : Inport  Port=2
  Vc1 : Inport  Port=3
  Iabc : Inport  Port=4
  Action Port : ActionPort  ActionPortLabel=if(u1 > 0.5)
  Abs3 : Abs
  Abs4 : Abs
  Abs5 : Abs
  Demux : Demux  Outputs=3
  Gain : Gain  Gain=1/5
  MATLAB Function1 : MATLAB Function  TreatAsAtomicUnit=on
  Max1 : MinMax  Function=max  Inputs=3
  Sum1 : Sum  Inputs=|-+
  V1 : Outport
  wires:
  Abs3/1 -> Max1/1
  MATLAB Function1/2(y) -> Sum1/2
  Gain/1 -> Demux/1
  MATLAB Function1/1(x) -> Sum1/1
  Abs4/1 -> Max1/2
  Abs5/1 -> Max1/3
  Max1/1 -> MATLAB Function1/7(max_i)  "max_i"
  Demux/3 -> MATLAB Function1/6(ic), Abs5/1
  Demux/2 -> MATLAB Function1/5(ib), Abs4/1
  Demux/1 -> MATLAB Function1/4(ia), Abs3/1
  Sum1/1 -> V1/1  "zero_seq"
  Va1/1 -> MATLAB Function1/1(va)
  Vb1/1 -> MATLAB Function1/2(vb)
  Vc1/1 -> MATLAB Function1/3(vc)
  Iabc/1 -> Gain/1

== matlab function FieldControl_PID/Field_control_PID/Current_control/SVM-DPWM/Variant Subsystem/DPWM/MATLAB Function1 ==
  data: x output; y output; va input; vb input; vc input; ia input; ib input; ic input; max_i input
function [x,y]= fcn(va,vb,vc,ia,ib,ic,max_i)

if (ia/max_i) == 1 || (ia/max_i) == -1
    y = va/abs(va); %get the sign of va
    x = va;
elseif (ib/max_i) == 1 || (ib/max_i) == -1
    y = vb/abs(vb);
    x = vb;
elseif (ic/max_i) == 1|| (ic/max_i) == -1
    y = vc/abs(vc);
    x = vc;
else
    y = NaN;
    x = NaN;
end

== matlab function FieldControl_PID/Field_control_PID/Speed_control/SVM-DPWM1/Variant Subsystem/Auto/If Action Subsystem1/MATLAB Function1 ==
  data: x output; y output; va input; vb input; vc input; ia input; ib input; ic input; max_i input
function [x,y]= fcn(va,vb,vc,ia,ib,ic,max_i)

if (ia/max_i) == 1 || (ia/max_i) == -1
    y = va/abs(va); %get the sign of va
    x = va;
elseif (ib/max_i) == 1 || (ib/max_i) == -1
    y = vb/abs(vb);
    x = vb;
elseif (ic/max_i) == 1|| (ic/max_i) == -1
    y = vc/abs(vc);
    x = vc;
else
    y = NaN;
    x = NaN;
end

== matlab function FieldControl_PID/Field_control_PID/Speed_control/SVM-DPWM1/Variant Subsystem/DPWM/MATLAB Function1 ==
  data: x output; y output; va input; vb input; vc input; ia input; ib input; ic input; max_i input
function [x,y]= fcn(va,vb,vc,ia,ib,ic,max_i)

if (ia/max_i) == 1 || (ia/max_i) == -1
    y = va/abs(va); %get the sign of va
    x = va;
elseif (ib/max_i) == 1 || (ib/max_i) == -1
    y = vb/abs(vb);
    x = vb;
elseif (ic/max_i) == 1|| (ic/max_i) == -1
    y = vc/abs(vc);
    x = vc;
else
    y = NaN;
    x = NaN;
end

== stateflow chart FieldControl_PID/Field_control_PID/Current_control/Switching_Frequency/Chart ==
  state Start
    state In_range
      du:
      Sampling_Mode=2;
      Fsw_out=Fsw_input;
    state Very_lower_Range
      en:
      Sampling_Mode=1;
      du:
      Fsw_out=Low_limit;
    state Lower_Range
      en:
      Sampling_Mode=1;
      du:
      Fsw_out=2*Fsw_input;
    state Higher_Range
      en:
      Sampling_Mode=2;
      du:
      Fsw_out=High_Limit;
    (default) -> In_range
    In_range -> Very_lower_Range [order 3] : [Fsw_input<Low_limit && Fsw_input <=Vlow_limit]{Fsw_out=Low_limit;}
    Very_lower_Range -> (junction 17) [order 1] : [Fsw_input>=Low_limit && Fsw_input <=High_Limit]
    Very_lower_Range -> Lower_Range [order 2] : [Fsw_input<Low_limit && Fsw_input >Vlow_limit]{Fsw_out=Low_limit;}
    Lower_Range -> Very_lower_Range [order 2] : [Fsw_input<Low_limit && Fsw_input <=Vlow_limit]{Fsw_out=Low_limit;}
    Higher_Range -> Very_lower_Range [order 3] : [Fsw_input<Low_limit && Fsw_input <=Vlow_limit]{Fsw_out=Low_limit;}
    Very_lower_Range -> Higher_Range [order 3] : [Fsw_input>High_Limit ]{Fsw_out=High_Limit;}
    Lower_Range -> (junction 17) [order 1] : [Fsw_input>=Low_limit && Fsw_input <=High_Limit]
    (junction 17) -> In_range : {Fsw_out=Fsw_input;}
    Higher_Range -> (junction 17) [order 1] : [Fsw_input>=Low_limit && Fsw_input <=High_Limit]
    In_range -> Lower_Range [order 2] : [Fsw_input<Low_limit && Fsw_input >Vlow_limit]{Fsw_out=2*Fsw_input;}
    Lower_Range -> Higher_Range [order 3] : [Fsw_input>High_Limit ]{Fsw_out=High_Limit;}
    Higher_Range -> Lower_Range [order 2] : [Fsw_input<Low_limit && Fsw_input >Vlow_limit]{Fsw_out=Low_limit;}
    In_range -> Higher_Range [order 1] : [Fsw_input>High_Limit ]{Fsw_out=High_Limit;}
  (default) -> Start
  data: Low_limit input; High_Limit input; Fsw_input input; Fsw_out output double; Sampling_Mode output double; Vlow_limit local double =2000

== matlab function FieldControl_PID/Field_control_PID/Current_control/SVM-DPWM/Variant Subsystem/Auto/If Action Subsystem1/MATLAB Function1 ==
  data: x output; y output; va input; vb input; vc input; ia input; ib input; ic input; max_i input
function [x,y]= fcn(va,vb,vc,ia,ib,ic,max_i)

if (ia/max_i) == 1 || (ia/max_i) == -1
    y = va/abs(va); %get the sign of va
    x = va;
elseif (ib/max_i) == 1 || (ib/max_i) == -1
    y = vb/abs(vb);
    x = vb;
elseif (ic/max_i) == 1|| (ic/max_i) == -1
    y = vc/abs(vc);
    x = vc;
else
    y = NaN;
    x = NaN;
end

== stateflow chart FieldControl_PID/Field_control_PID/Speed_control/Triggered Speed_Control/Switching_Frequency/Chart ==
  state Start
    state In_range
      du:
      Sampling_Mode=2;
      Fsw_out=Fsw_input;
    state Very_lower_Range
      en:
      Sampling_Mode=1;
      du:
      Fsw_out=Low_limit;
    state Lower_Range
      en:
      Sampling_Mode=1;
      du:
      Fsw_out=2*Fsw_input;
    state Higher_Range
      en:
      Sampling_Mode=2;
      du:
      Fsw_out=High_Limit;
    (default) -> In_range
    In_range -> Very_lower_Range [order 3] : [Fsw_input<Low_limit && Fsw_input <=Vlow_limit]{Fsw_out=Low_limit;}
    Very_lower_Range -> (junction 17) [order 1] : [Fsw_input>=Low_limit && Fsw_input <=High_Limit]
    Very_lower_Range -> Lower_Range [order 2] : [Fsw_input<Low_limit && Fsw_input >Vlow_limit]{Fsw_out=Low_limit;}
    Lower_Range -> Very_lower_Range [order 2] : [Fsw_input<Low_limit && Fsw_input <=Vlow_limit]{Fsw_out=Low_limit;}
    Higher_Range -> Very_lower_Range [order 3] : [Fsw_input<Low_limit && Fsw_input <=Vlow_limit]{Fsw_out=Low_limit;}
    Very_lower_Range -> Higher_Range [order 3] : [Fsw_input>High_Limit ]{Fsw_out=High_Limit;}
    Lower_Range -> (junction 17) [order 1] : [Fsw_input>=Low_limit && Fsw_input <=High_Limit]
    (junction 17) -> In_range : {Fsw_out=Fsw_input;}
    Higher_Range -> (junction 17) [order 1] : [Fsw_input>=Low_limit && Fsw_input <=High_Limit]
    In_range -> Lower_Range [order 2] : [Fsw_input<Low_limit && Fsw_input >Vlow_limit]{Fsw_out=2*Fsw_input;}
    Lower_Range -> Higher_Range [order 3] : [Fsw_input>High_Limit ]{Fsw_out=High_Limit;}
    Higher_Range -> Lower_Range [order 2] : [Fsw_input<Low_limit && Fsw_input >Vlow_limit]{Fsw_out=Low_limit;}
    In_range -> Higher_Range [order 1] : [Fsw_input>High_Limit ]{Fsw_out=High_Limit;}
  (default) -> Start
  data: Low_limit input; High_Limit input; Fsw_input input; Fsw_out output double; Sampling_Mode output double; Vlow_limit local double =2000
